simulink model "RPPPWM"  (R2014a)
settings: Solver=ode113  StartTime=0.0  StopTime=8  RelTol=1e-3
undefined symbols (not defined in the file): J, p, Rr, Rs, wb, Xlr, Xls, Xmstar
libraries: powerlib x16, simulink_extras x9, powerlib_extras x1
settings Model: Creator=afroz khan  LastModifiedBy=Divya M

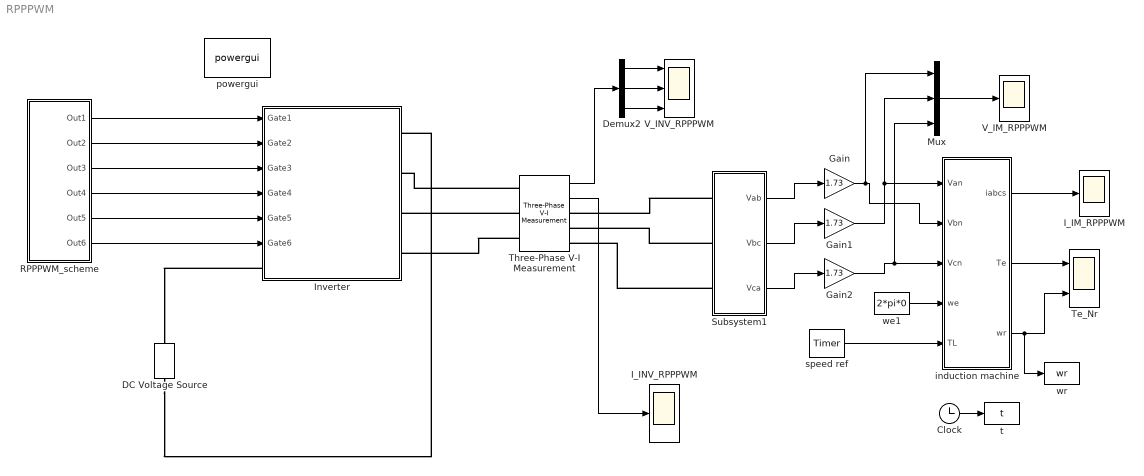
== system RPPPWM ==
  Clock : Clock
  DC Voltage Source : powerlib/Electrical Sources/DC Voltage Source  Amplitude=400  Measurements=None
  Demux2 : Demux  Outputs=3
  Gain : Gain  Gain=1.73
  Gain1 : Gain  Gain=1.73
  Gain2 : Gain  Gain=1.73
  I_IM_RPPPWM : Scope
      settings: YMin=-80  YMax=70  SaveName=I_IM_RPPPWM  MaxDataPoints=50000
  I_INV_RPPPWM : Scope
      settings: YMin=-75  YMax=75  SaveName=I_INV_RPPPWM  MaxDataPoints=50000
  Inverter : Subsystem
  Mux : Mux  Inputs=3
  RPPPWM_scheme : Subsystem
  Subsystem1 : Subsystem
  Te_Nr : Scope  NumInputPorts=2
      settings: TimeRange=1.5  YMin=-35~265  YMax=75~315  SaveName=ScopeData2
  Three-Phase V-I Measurement : powerlib/Measurements/Three-Phase V-I Measurement  VoltageMeasurement=phase-to-phase  SetLabelV=off  LabelV=Vabc  Vpu=off  VpuLL=off  CurrentMeasurement=yes  SetLabelI=off  LabelI=Iabc  Ipu=off  Pbase=100e6  Vbase=500e3  OutputType=Complex  PhasorSimulation=off  PSBequivalent=0
  V_IM_RPPPWM : Scope
      settings: YMin=-700  YMax=700  SaveName=V_IM_RPPPWM  MaxDataPoints=50000
  V_INV_RPPPWM : Scope  NumInputPorts=3
      settings: YMin=-225~-5~-5  YMax=225~5~5  SaveName=V_INV_RPPPWM  MaxDataPoints=50000
  "induction machine " : Subsystem
  powergui : powerlib/powergui  Priority=1  SimulationMode=Discrete  SolverType=Tustin  SampleTime=50e-6  frequency=60  SPID=off  DisableSnubberDevices=off  DisableRonSwitches=off  DisableVfSwitches=off  SwTol=0  Interpol=off  DisplayEquations=off  Ts=0  methode=off  frequencyindice=0  Pbase=100e6  ErrMax=1e-4  Iterations=50  UnitsV=kV  UnitsW=MW  FunctionMessages=off  echomessages=off  HookPort=off  EnableUseOfTLC=off  x0status=blocks  RestoreLinks=warning  ResistiveCurrentMeasurement=off  Frange=[0:2:500]  Ylog=off  Xlog=on  ShowGrid=off  save=off  variable=ZData  structure=V_IM_RPPPWM  ZoomFFT=off  StartTime=7.5  cycles=10  DisplayStyle=1  fundamental=50  FreqAxis=off  MaxFrequency=5000  frequencyindicesteady=1  RmsSteady=1  display=off
  speed ref : powerlib_extras/Control  Blocks/Timer  t=[ 0 1]  e=[10 10]
  t : ToWorkspace  VariableName=t  SampleTime=-1
  we1 : Constant  Value=2*pi*0
  wr : ToWorkspace  VariableName=wr  SampleTime=-1
  wires:
  RPPPWM_scheme/1(Out1) -> Inverter/1(Gate1)
  RPPPWM_scheme/2(Out2) -> Inverter/2(Gate2)
  RPPPWM_scheme/3(Out3) -> Inverter/3(Gate3)
  RPPPWM_scheme/4(Out4) -> Inverter/4(Gate4)
  RPPPWM_scheme/5(Out5) -> Inverter/5(Gate5)
  RPPPWM_scheme/6(Out6) -> Inverter/6(Gate6)
  Demux2/1 -> V_INV_RPPPWM/1
  Demux2/2 -> V_INV_RPPPWM/2
  Demux2/3 -> V_INV_RPPPWM/3
  Three-Phase V-I Measurement/1 -> Demux2/1
  Gain2/1 -> "induction machine "/3(Vcn), Mux/3
  Subsystem1/3(Vca) -> Gain2/1
  Gain1/1 -> "induction machine "/1(Van), Mux/2
  Gain/1 -> "induction machine "/2(Vbn), Mux/1
  Subsystem1/2(Vbc) -> Gain1/1
  Subsystem1/1(Vab) -> Gain/1
  Mux/1 -> V_IM_RPPPWM/1
  speed ref/1 -> "induction machine "/5(TL)
  we1/1 -> "induction machine "/4(we)
  "induction machine "/2(Te) -> Te_Nr/1
  "induction machine "/3(wr) -> wr/1, Te_Nr/2
  "induction machine "/1(iabcs) -> I_IM_RPPPWM/1
  Clock/1 -> t/1
  Three-Phase V-I Measurement/2 -> I_INV_RPPPWM/1
  connections:
  Inverter/LConn1 -- DC Voltage Source/RConn1
  DC Voltage Source/LConn1 -- Inverter/RConn1
  Three-Phase V-I Measurement/LConn1 -- Inverter/RConn2
  Three-Phase V-I Measurement/LConn2 -- Inverter/RConn3
  Three-Phase V-I Measurement/LConn3 -- Inverter/RConn4
  Subsystem1/LConn1 -- Three-Phase V-I Measurement/RConn1
  Subsystem1/LConn2 -- Three-Phase V-I Measurement/RConn2
  Subsystem1/LConn3 -- Three-Phase V-I Measurement/RConn3

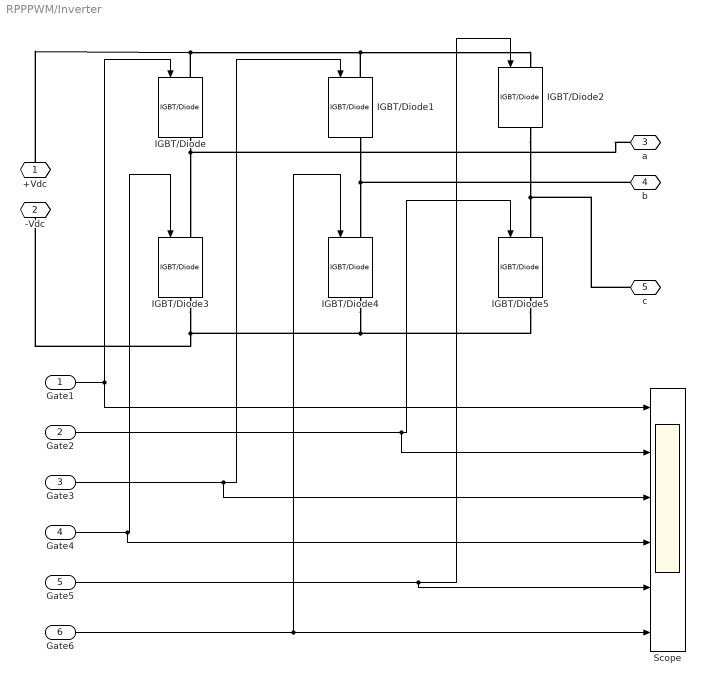
== system RPPPWM/Inverter ==
  Gate1 : Inport
  Gate2 : Inport  Port=2
  Gate3 : Inport  Port=3
  Gate4 : Inport  Port=4
  Gate5 : Inport  Port=5
  Gate6 : Inport  Port=6
  IGBT/Diode{,1..5} (6 alike) : powerlib/Power Electronics/IGBT//Diode  Ron=1e-3  Rs=1e5  Cs=inf  Measurements=on
  Scope : Scope  NumInputPorts=6
      settings: YMin=-5~-5~-5~-5~-5~-5  YMax=5~5~5~5~5~5
  +Vdc : PMIOPort  Port=1  Side=Left
  -Vdc : PMIOPort  Port=2  Side=Right
  a : PMIOPort  Port=3  Side=Right
  b : PMIOPort  Port=4  Side=Right
  c : PMIOPort  Port=5  Side=Right
  wires:
  Gate2/1 -> Scope/2, IGBT/Diode5/1
  Gate3/1 -> Scope/3, IGBT/Diode1/1
  Gate4/1 -> Scope/4, IGBT/Diode3/1
  Gate6/1 -> IGBT/Diode4/1, Scope/6
  Gate1/1 -> IGBT/Diode/1, Scope/1
  Gate5/1 -> Scope/5, IGBT/Diode2/1
  connections:
  IGBT/Diode5/RConn1 -- IGBT/Diode4/RConn1 -- -Vdc/RConn1 -- IGBT/Diode3/RConn1
  IGBT/Diode2/RConn1 -- c/RConn1 -- IGBT/Diode5/LConn1
  IGBT/Diode1/RConn1 -- b/RConn1 -- IGBT/Diode4/LConn1
  IGBT/Diode/LConn1 -- +Vdc/RConn1 -- IGBT/Diode1/LConn1 -- IGBT/Diode2/LConn1
  IGBT/Diode/RConn1 -- a/RConn1 -- IGBT/Diode3/LConn1

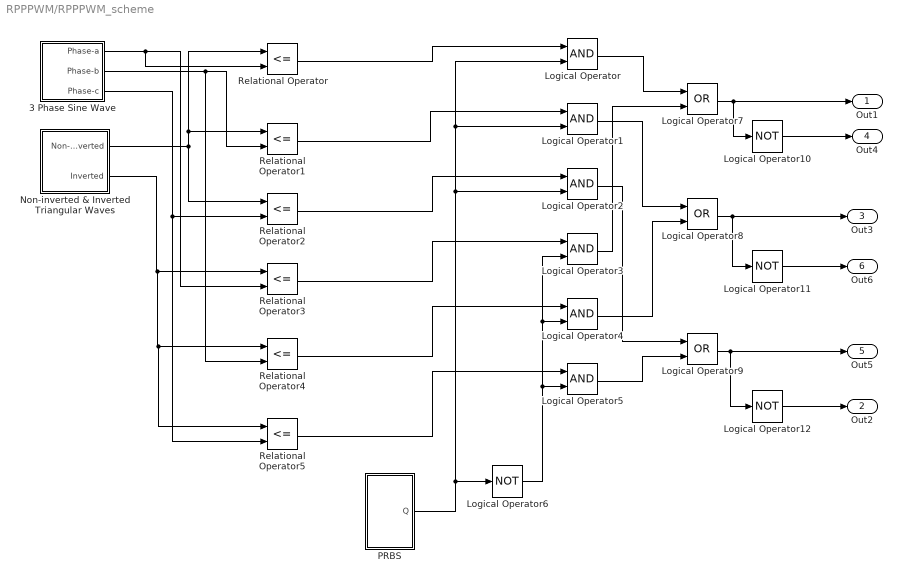
== system RPPPWM/RPPPWM_scheme ==
  3 Phase Sine Wave : Subsystem
  Logical Operator{,1..5} (6 alike) : Logic  AllPortsSameDT=off  OutDataTypeStr=boolean
  Logical Operator{6,10..12} (4 alike) : Logic  Operator=NOT  AllPortsSameDT=off  OutDataTypeStr=boolean
  Logical Operator7 : Logic  Operator=OR  AllPortsSameDT=off  OutDataTypeStr=boolean
  Logical Operator8 : Logic  Operator=OR  AllPortsSameDT=off  OutDataTypeStr=boolean
  Logical Operator9 : Logic  Operator=OR  AllPortsSameDT=off  OutDataTypeStr=boolean
  Non-inverted & Inverted Triangular Waves : Subsystem
  PRBS : Subsystem
  Relational Operator{,1..5} (6 alike) : RelationalOperator  Operator=<=  OutDataTypeStr=boolean
  Out1 : Outport
  Out2 : Outport  Port=2
  Out3 : Outport  Port=3
  Out4 : Outport  Port=4
  Out5 : Outport  Port=5
  Out6 : Outport  Port=6
  wires:
  Non-inverted & Inverted Triangular Waves/1(Non-inverted) -> Relational Operator2/1, Relational Operator1/1, Relational Operator/1
  Non-inverted & Inverted Triangular Waves/2(Inverted) -> Relational Operator5/1, Relational Operator4/1, Relational Operator3/1
  3 Phase Sine Wave/1("\tPhase-a") -> Relational Operator3/2, Relational Operator/2
  3 Phase Sine Wave/2(Phase-b) -> Relational Operator4/2, Relational Operator1/2
  3 Phase Sine Wave/3(Phase-c) -> Relational Operator5/2, Relational Operator2/2
  Relational Operator/1 -> Logical Operator/1
  Relational Operator1/1 -> Logical Operator1/1
  Relational Operator2/1 -> Logical Operator2/1
  Relational Operator3/1 -> Logical Operator3/1
  Relational Operator4/1 -> Logical Operator4/1
  Relational Operator5/1 -> Logical Operator5/1
  PRBS/1(Q) -> Logical Operator6/1, Logical Operator2/2, Logical Operator1/2, Logical Operator/2
  Logical Operator6/1 -> Logical Operator5/2, Logical Operator4/2, Logical Operator3/2
  Logical Operator/1 -> Logical Operator7/1
  Logical Operator1/1 -> Logical Operator8/1
  Logical Operator2/1 -> Logical Operator9/1
  Logical Operator3/1 -> Logical Operator7/2
  Logical Operator4/1 -> Logical Operator8/2
  Logical Operator5/1 -> Logical Operator9/2
  Logical Operator7/1 -> Logical Operator10/1, Out1/1
  Logical Operator8/1 -> Logical Operator11/1, Out3/1
  Logical Operator9/1 -> Logical Operator12/1, Out5/1
  Logical Operator10/1 -> Out4/1
  Logical Operator11/1 -> Out6/1
  Logical Operator12/1 -> Out2/1

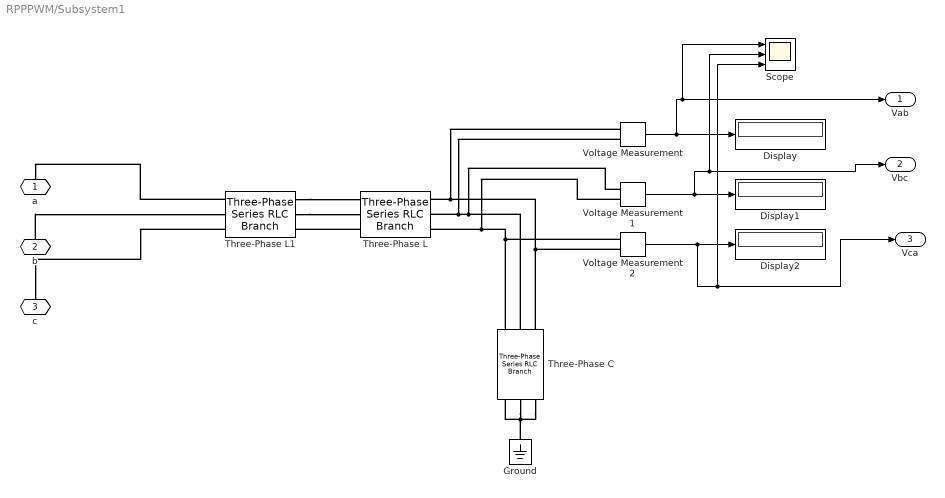
== system RPPPWM/Subsystem1 ==
  Display : Display
  Display1 : Display
  Display2 : Display
  Ground : powerlib/Elements/Ground  LConnTagsString=a
  Scope : Scope  NumInputPorts=3
      settings: YMin=-200~-200~-200  YMax=200~200~200  SaveName=ScopeData3
  "Three-Phase C " : powerlib/Elements/Three-Phase Series RLC Branch  LConnTagsString=A|B|C  RConnTagsString=A|B|C  BranchType=C  Resistance=1  Inductance=10  Capacitance=0.2420e-3  Measurements=None
  Three-Phase L : powerlib/Elements/Three-Phase Series RLC Branch  LConnTagsString=A|B|C  RConnTagsString=A|B|C  BranchType=L  Resistance=1  Inductance=0.0150e-2  Capacitance=1e-6  Measurements=None
  Three-Phase L1 : powerlib/Elements/Three-Phase Series RLC Branch  LConnTagsString=A|B|C  RConnTagsString=A|B|C  BranchType=R  Resistance=15  Inductance=1e-1  Capacitance=1e-6  Measurements=None
  Voltage Measurement : powerlib/Measurements/Voltage Measurement  PhasorSimulation=off  OutputType=Complex  PSBequivalent=0
  Voltage Measurement1 : powerlib/Measurements/Voltage Measurement  PhasorSimulation=off  OutputType=Complex  PSBequivalent=0
  Voltage Measurement2 : powerlib/Measurements/Voltage Measurement  PhasorSimulation=off  OutputType=Complex  PSBequivalent=0
  a : PMIOPort  Port=1  Side=Left
  b : PMIOPort  Port=2  Side=Left
  c : PMIOPort  Port=3  Side=Left
  Vab : Outport
  Vbc : Outport  Port=2
  Vca : Outport  Port=3
  wires:
  Voltage Measurement/1 -> Scope/1, Vab/1, Display/1
  Voltage Measurement1/1 -> Scope/2, Vbc/1, Display1/1
  Voltage Measurement2/1 -> Scope/3, Vca/1, Display2/1
  connections:
  "Three-Phase C "/LConn1 -- Voltage Measurement2/LConn1 -- Voltage Measurement1/LConn2 -- Three-Phase L/RConn3
  "Three-Phase C "/LConn2 -- Voltage Measurement1/LConn1 -- Voltage Measurement/LConn2 -- Three-Phase L/RConn2
  "Three-Phase C "/LConn3 -- Voltage Measurement2/LConn2 -- Voltage Measurement/LConn1 -- Three-Phase L/RConn1
  Ground/LConn1 -- "Three-Phase C "/RConn2 -- "Three-Phase C "/RConn1 -- "Three-Phase C "/RConn3
  Three-Phase L1/RConn1 -- Three-Phase L/LConn1
  Three-Phase L1/RConn2 -- Three-Phase L/LConn2
  Three-Phase L/LConn3 -- Three-Phase L1/RConn3
  Three-Phase L1/LConn1 -- a/RConn1
  b/RConn1 -- Three-Phase L1/LConn2
  Three-Phase L1/LConn3 -- c/RConn1

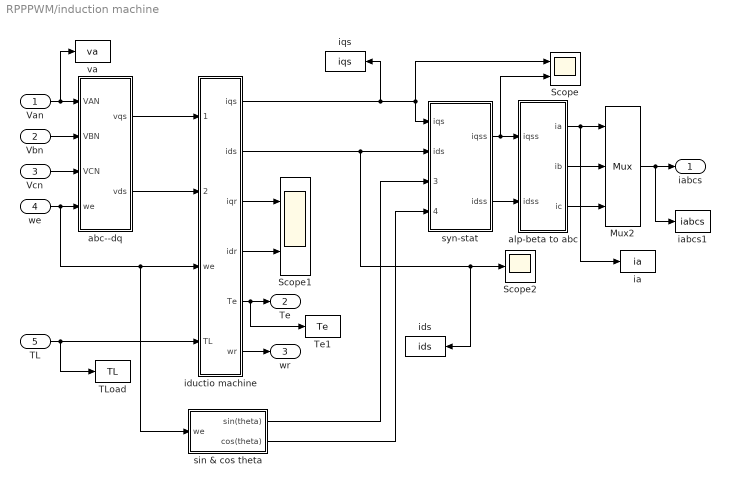
== system RPPPWM/induction machine  ==
  Van : Inport
  Vbn : Inport  Port=2
  Vcn : Inport  Port=3
  we : Inport  Port=4
  TL : Inport  Port=5
  " alp-beta to abc" : Subsystem
  Mux2 : Mux  Inputs=3
  Scope : Scope  NumInputPorts=2
      settings: YMin=-60~-5  YMax=50~5  SaveName=ScopeData11
  Scope1 : Scope  NumInputPorts=2
      settings: TimeRange=0.25  YMin=-350~-5  YMax=350~5  SampleInput=on
  Scope2 : Scope
      settings: YMin=-60  YMax=50  SaveName=ScopeData12
  TLoad : ToWorkspace  VariableName=TL  SampleTime=-1
  Te1 : ToWorkspace  VariableName=Te  SampleTime=-1
  "abc--dq " : Subsystem
  ia : ToWorkspace  VariableName=ia  SampleTime=-1
  iabcs1 : ToWorkspace  VariableName=iabcs  SampleTime=-1
  ids : ToWorkspace  VariableName=ids  SampleTime=-1
  iductio machine : Subsystem
  iqs : ToWorkspace  VariableName=iqs  SampleTime=-1
  sin & cos theta : Subsystem
  syn-stat : Subsystem
  va : ToWorkspace  VariableName=va  SampleTime=-1
  iabcs : Outport
  Te : Outport  Port=2
  wr : Outport  Port=3
  wires:
  Van/1 -> "abc--dq "/1(VAN), va/1
  Vbn/1 -> "abc--dq "/2(VBN)
  Vcn/1 -> "abc--dq "/3(VCN)
  we/1 -> sin & cos theta/1(we), iductio machine/3(we), "abc--dq "/4(we)
  TL/1 -> iductio machine/4(TL), TLoad/1
  iductio machine/4(idr) -> Scope1/2
  iductio machine/3(iqr) -> Scope1/1
  sin & cos theta/2(cos(theta)) -> syn-stat/4(cos(theta))
  sin & cos theta/1(sin(theta)) -> syn-stat/3(sin(theta))
  " alp-beta to abc"/3(ic) -> Mux2/3
  " alp-beta to abc"/2(ib) -> Mux2/2
  syn-stat/2(idss) -> " alp-beta to abc"/2(idss)
  syn-stat/1(iqss) -> " alp-beta to abc"/1(iqss), Scope/2
  iductio machine/1(iqs) -> syn-stat/1(iqs), Scope/1, iqs/1
  "abc--dq "/2(vds) -> iductio machine/2(vds)
  "abc--dq "/1(vqs) -> iductio machine/1(vqs)
  iductio machine/5(Te) -> Te/1, Te1/1
  iductio machine/2(ids) -> syn-stat/2(ids), Scope2/1, ids/1
  " alp-beta to abc"/1(ia) -> Mux2/1, ia/1
  Mux2/1 -> iabcs/1, iabcs1/1
  iductio machine/6(wr) -> wr/1

== system RPPPWM/RPPPWM_scheme/3 Phase Sine Wave ==
  Scope : Scope  NumInputPorts=3
      settings: YMin=-5~-5~-5  YMax=5~5~5  SaveName=ScopeData9
  Sine Wave : Sin  Amplitude=0.8  Frequency=314  SampleTime=0
  Sine Wave1 : Sin  Amplitude=0.8  Frequency=314  Phase=(2*pi)/3  SampleTime=0
  Sine Wave2 : Sin  Amplitude=0.8  Frequency=314  Phase=(4*pi)/3  SampleTime=0
  "\tPhase-a" : Outport
  Phase-b : Outport  Port=2
  Phase-c : Outport  Port=3
  wires:
  Sine Wave1/1 -> Scope/2, Phase-b/1
  Sine Wave/1 -> Scope/1, "\tPhase-a"/1
  Sine Wave2/1 -> Scope/3, Phase-c/1

== system RPPPWM/RPPPWM_scheme/Non-inverted & Inverted Triangular Waves ==
  note: Triangular Wave
  Constant : Constant  Value=-1
  Dot Product : DotProduct  InputSameDT=on  OutDataTypeStr=Inherit: Inherit via internal rule
  Integrator : Integrator
  Pulse Generator : DiscretePulseGenerator  PulseType=Time based  Amplitude=12000  Period=1e-3/3  PulseWidth=50
  Pulse Generator1 : DiscretePulseGenerator  PulseType=Time based  Amplitude=-12000  Period=1/3e3  PulseWidth=50  PhaseDelay=1/6e3
  Scope : Scope  NumInputPorts=2
      settings: YMin=-2.5~-37.5  YMax=37.5~2.5  SaveName=ScopeData6
  Sum : Sum  Inputs=|++
  Sum1 : Sum  Inputs=|++
  Non-inverted : Outport
  Inverted : Outport  Port=2
  wires:
  Dot Product/1 -> Scope/2, Inverted/1  "Inverted Triangular Wave"
  Pulse Generator/1 -> Sum/1
  Pulse Generator1/1 -> Sum/2
  Sum/1 -> Integrator/1
  Sum1/1 -> Scope/1, Non-inverted/1, Dot Product/1
  Constant/1 -> Dot Product/2, Sum1/2
  Integrator/1 -> Sum1/1

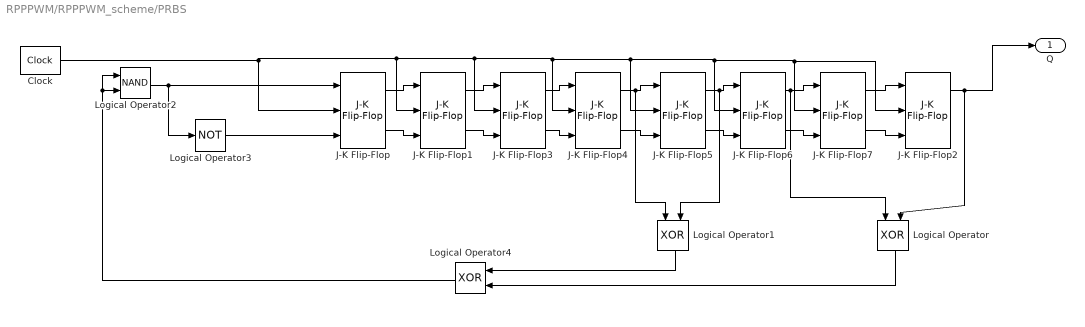
== system RPPPWM/RPPPWM_scheme/PRBS ==
  Clock : simulink_extras/Flip Flops/Clock  period=1/3e3
  J-K Flip-Flop{,1..7} (8 alike) : simulink_extras/Flip Flops/J-K Flip-Flop  initial_condition=0
  Logical Operator : Logic  Operator=XOR  AllPortsSameDT=off  OutDataTypeStr=boolean
  Logical Operator1 : Logic  Operator=XOR  AllPortsSameDT=off  OutDataTypeStr=boolean
  Logical Operator2 : Logic  Operator=NAND  AllPortsSameDT=off  OutDataTypeStr=boolean
  Logical Operator3 : Logic  Operator=NOT  AllPortsSameDT=off  OutDataTypeStr=boolean
  Logical Operator4 : Logic  Operator=XOR  AllPortsSameDT=off  OutDataTypeStr=boolean
  Q : Outport
  wires:
  J-K Flip-Flop6/1 -> Logical Operator/1, J-K Flip-Flop7/1
  Logical Operator2/1 -> Logical Operator3/1, J-K Flip-Flop/1
  J-K Flip-Flop5/2 -> J-K Flip-Flop6/3
  J-K Flip-Flop3/2 -> J-K Flip-Flop4/3
  Logical Operator/1 -> Logical Operator4/2
  J-K Flip-Flop7/1 -> J-K Flip-Flop2/1
  J-K Flip-Flop5/1 -> J-K Flip-Flop6/1, Logical Operator1/2
  Logical Operator1/1 -> Logical Operator4/1
  J-K Flip-Flop1/2 -> J-K Flip-Flop3/3
  J-K Flip-Flop/2 -> J-K Flip-Flop1/3
  Logical Operator4/1 -> Logical Operator2/2, Logical Operator2/1
  J-K Flip-Flop3/1 -> J-K Flip-Flop4/1
  J-K Flip-Flop4/1 -> J-K Flip-Flop5/1, Logical Operator1/1
  J-K Flip-Flop7/2 -> J-K Flip-Flop2/3
  J-K Flip-Flop6/2 -> J-K Flip-Flop7/3
  J-K Flip-Flop2/1 -> Q/1, Logical Operator/2
  Logical Operator3/1 -> J-K Flip-Flop/3
  Clock/1 -> J-K Flip-Flop3/2, J-K Flip-Flop2/2, J-K Flip-Flop7/2, J-K Flip-Flop6/2, J-K Flip-Flop5/2, J-K Flip-Flop4/2, J-K Flip-Flop1/2, J-K Flip-Flop/2
  J-K Flip-Flop4/2 -> J-K Flip-Flop5/3
  J-K Flip-Flop/1 -> J-K Flip-Flop1/1
  J-K Flip-Flop1/1 -> J-K Flip-Flop3/1

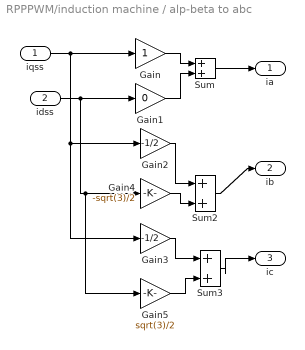
== system RPPPWM/induction machine / alp-beta to abc ==
  iqss : Inport
  idss : Inport  Port=2
  Gain : Gain  SaturateOnIntegerOverflow=on  OutDataTypeStr=Inherit: Same as input  ParamDataTypeStr=Inherit: Same as input
  Gain1 : Gain  Gain=0  SaturateOnIntegerOverflow=on  OutDataTypeStr=Inherit: Same as input  ParamDataTypeStr=Inherit: Same as input
  Gain2 : Gain  Gain=-1/2  SaturateOnIntegerOverflow=on  OutDataTypeStr=Inherit: Same as input  ParamDataTypeStr=Inherit: Same as input
  Gain3 : Gain  Gain=-1/2  SaturateOnIntegerOverflow=on  OutDataTypeStr=Inherit: Same as input  ParamDataTypeStr=Inherit: Same as input
  Gain4 : Gain  Gain=-sqrt(3)/2  SaturateOnIntegerOverflow=on  OutDataTypeStr=Inherit: Same as input  ParamDataTypeStr=Inherit: Same as input
  Gain5 : Gain  Gain=sqrt(3)/2  SaturateOnIntegerOverflow=on  OutDataTypeStr=Inherit: Same as input  ParamDataTypeStr=Inherit: Same as input
  Sum : Sum  Inputs=|++  SaturateOnIntegerOverflow=on
  Sum2 : Sum  Inputs=|++  SaturateOnIntegerOverflow=on
  Sum3 : Sum  Inputs=|++  SaturateOnIntegerOverflow=on
  ia : Outport
  ib : Outport  Port=2
  ic : Outport  Port=3
  wires:
  Gain/1 -> Sum/1
  Gain1/1 -> Sum/2
  Gain2/1 -> Sum2/1
  Gain4/1 -> Sum2/2
  Gain3/1 -> Sum3/1
  Gain5/1 -> Sum3/2
  iqss/1 -> Gain3/1, Gain2/1, Gain/1
  idss/1 -> Gain5/1, Gain4/1, Gain1/1
  Sum3/1 -> ic/1
  Sum2/1 -> ib/1
  Sum/1 -> ia/1

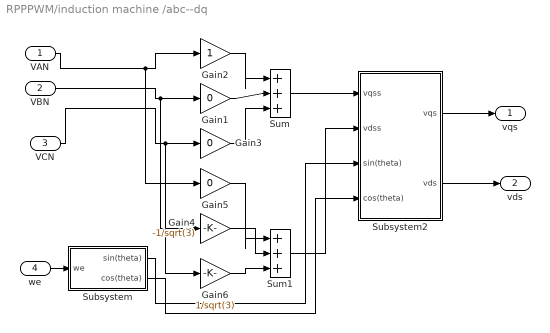
== system RPPPWM/induction machine /abc--dq  ==
  VAN : Inport
  VBN : Inport  Port=2
  VCN : Inport  Port=3
  we : Inport  Port=4
  Gain1 : Gain  Gain=0  SaturateOnIntegerOverflow=on  OutDataTypeStr=Inherit: Same as input  ParamDataTypeStr=Inherit: Same as input
  Gain2 : Gain  SaturateOnIntegerOverflow=on  OutDataTypeStr=Inherit: Same as input  ParamDataTypeStr=Inherit: Same as input
  Gain3 : Gain  Gain=0  SaturateOnIntegerOverflow=on  OutDataTypeStr=Inherit: Same as input  ParamDataTypeStr=Inherit: Same as input
  Gain4 : Gain  Gain=-1/sqrt(3)  SaturateOnIntegerOverflow=on  OutDataTypeStr=Inherit: Same as input  ParamDataTypeStr=Inherit: Same as input
  Gain5 : Gain  Gain=0  SaturateOnIntegerOverflow=on  OutDataTypeStr=Inherit: Same as input  ParamDataTypeStr=Inherit: Same as input
  Gain6 : Gain  Gain=1/sqrt(3)  SaturateOnIntegerOverflow=on  OutDataTypeStr=Inherit: Same as input  ParamDataTypeStr=Inherit: Same as input
  Subsystem : Subsystem
  Subsystem2 : Subsystem
  Sum : Sum  Inputs=|+++  SaturateOnIntegerOverflow=on
  Sum1 : Sum  Inputs=|+++  SaturateOnIntegerOverflow=on
  vqs : Outport
  vds : Outport  Port=2
  wires:
  Gain2/1 -> Sum/1
  Gain1/1 -> Sum/2
  Gain3/1 -> Sum/3
  Gain5/1 -> Sum1/1
  Gain4/1 -> Sum1/2
  Gain6/1 -> Sum1/3
  Sum/1 -> Subsystem2/1(vqss)
  Sum1/1 -> Subsystem2/2(vdss)
  VAN/1 -> Gain2/1, Gain5/1
  VBN/1 -> Gain1/1, Gain4/1
  VCN/1 -> Gain3/1, Gain6/1
  Subsystem2/1(vqs) -> vqs/1
  Subsystem2/2(vds) -> vds/1
  we/1 -> Subsystem/1(we)
  Subsystem/1(sin(theta)) -> Subsystem2/3(sin(theta))
  Subsystem/2(cos(theta)) -> Subsystem2/4(cos(theta))

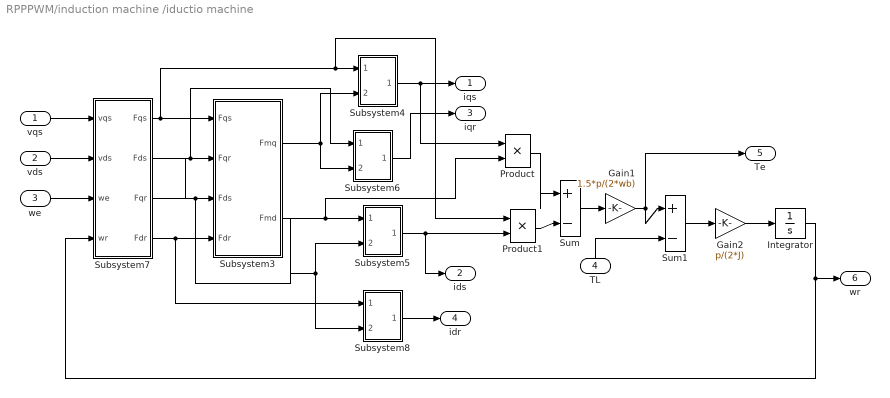
== system RPPPWM/induction machine /iductio machine ==
  vqs : Inport
  vds : Inport  Port=2
  we : Inport  Port=3
  TL : Inport  Port=4
  Gain1 : Gain  Gain=1.5*p/(2*wb)  SaturateOnIntegerOverflow=on  OutDataTypeStr=Inherit: Same as input  ParamDataTypeStr=Inherit: Same as input
  Gain2 : Gain  Gain=p/(2*J)  SaturateOnIntegerOverflow=on  OutDataTypeStr=Inherit: Same as input  ParamDataTypeStr=Inherit: Same as input
  Integrator : Integrator
  Product : Product  SaturateOnIntegerOverflow=on  OutDataTypeStr=Inherit: Same as first input
  Product1 : Product  SaturateOnIntegerOverflow=on  OutDataTypeStr=Inherit: Same as first input
  Subsystem3 : Subsystem
  Subsystem4 : Subsystem
  Subsystem5 : Subsystem
  Subsystem6 : Subsystem
  Subsystem7 : Subsystem
  Subsystem8 : Subsystem
  Sum : Sum  Inputs=|+-  SaturateOnIntegerOverflow=on
  Sum1 : Sum  Inputs=|+-  SaturateOnIntegerOverflow=on
  iqs : Outport
  ids : Outport  Port=2
  iqr : Outport  Port=3
  idr : Outport  Port=4
  Te : Outport  Port=5
  wr : Outport  Port=6
  wires:
  Subsystem7/1(Fqs) -> Subsystem3/1(Fqs), Subsystem4/1(Fqs), Product1/1
  Subsystem3/1(Fmq) -> Subsystem4/2(Fmq), Subsystem6/2(Fmq)
  Subsystem3/2(Fmd) -> Subsystem5/2(Fmd), Subsystem8/2(Fmd)
  Subsystem4/1(iqs) -> Product/1, iqs/1
  Subsystem5/1(ids) -> Product1/2, ids/1
  Sum/1 -> Gain1/1
  Gain1/1 -> Te/1, Sum1/1
  Gain2/1 -> Integrator/1
  Integrator/1 -> wr/1, Subsystem7/4(wr)
  we/1 -> Subsystem7/3(we)
  vqs/1 -> Subsystem7/1(vqs)
  vds/1 -> Subsystem7/2(vds)
  Subsystem6/1(iqr) -> iqr/1
  Subsystem8/1(idr) -> idr/1
  Product1/1 -> Sum/2
  Product/1 -> Sum/1
  Sum1/1 -> Gain2/1
  TL/1 -> Sum1/2
  Subsystem7/3(Fqr) -> Subsystem3/2(Fqr), Subsystem6/1(Fqr)
  Subsystem7/4(Fdr) -> Subsystem3/4(Fdr), Subsystem8/1(Fdr)
  Subsystem7/2(Fds) -> Subsystem3/3(Fds), Subsystem5/1(Fds), Product/2

== system RPPPWM/induction machine /sin & cos theta ==
  we : Inport
  Integrator : Integrator
  Trigonometric Function : Trigonometry
  Trigonometric Function1 : Trigonometry  Operator=cos
  sin(theta) : Outport
  cos(theta) : Outport  Port=2
  wires:
  Integrator/1 -> Trigonometric Function/1, Trigonometric Function1/1
  Trigonometric Function/1 -> sin(theta)/1
  we/1 -> Integrator/1
  Trigonometric Function1/1 -> cos(theta)/1

== system RPPPWM/induction machine /syn-stat ==
  iqs : Inport
  ids : Inport  Port=2
  sin(theta) : Inport  Port=3
  cos(theta) : Inport  Port=4
  Product{,1..3} (4 alike) : Product  SaturateOnIntegerOverflow=on  OutDataTypeStr=Inherit: Same as first input
  Sum1 : Sum  SaturateOnIntegerOverflow=on
  Sum4 : Sum  Inputs=-+  SaturateOnIntegerOverflow=on
  iqss : Outport
  idss : Outport  Port=2
  wires:
  ids/1 -> Product3/1, Product/1
  iqs/1 -> Product2/1, Product1/1
  Product1/1 -> Sum1/1
  Product/1 -> Sum1/2
  Product2/1 -> Sum4/1
  Product3/1 -> Sum4/2
  sin(theta)/1 -> Product/2, Product2/2
  cos(theta)/1 -> Product1/2, Product3/2
  Sum1/1 -> iqss/1
  Sum4/1 -> idss/1

== system RPPPWM/induction machine /abc--dq /Subsystem ==
  we : Inport
  Integrator : Integrator
  Trigonometric Function : Trigonometry
  Trigonometric Function1 : Trigonometry  Operator=cos
  sin(theta) : Outport
  cos(theta) : Outport  Port=2
  wires:
  Integrator/1 -> Trigonometric Function/1, Trigonometric Function1/1
  Trigonometric Function/1 -> sin(theta)/1
  we/1 -> Integrator/1
  Trigonometric Function1/1 -> cos(theta)/1

== system RPPPWM/induction machine /abc--dq /Subsystem2 ==
  vqss : Inport
  vdss : Inport  Port=2
  sin(theta) : Inport  Port=3
  cos(theta) : Inport  Port=4
  Product{,1..3} (4 alike) : Product  SaturateOnIntegerOverflow=on  OutDataTypeStr=Inherit: Same as first input
  Sum : Sum  Inputs=+-  SaturateOnIntegerOverflow=on
  Sum1 : Sum  SaturateOnIntegerOverflow=on
  vqs : Outport
  vds : Outport  Port=2
  wires:
  vqss/1 -> Product2/1, Product/1
  vdss/1 -> Product1/1, Product3/1
  sin(theta)/1 -> Product2/2, Product1/2
  Product/1 -> Sum/1
  Product1/1 -> Sum/2
  Product2/1 -> Sum1/1
  Product3/1 -> Sum1/2
  Sum/1 -> vqs/1
  Sum1/1 -> vds/1
  cos(theta)/1 -> Product3/2, Product/2

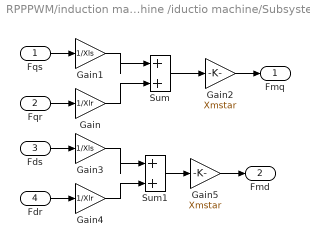
== system RPPPWM/induction machine /iductio machine/Subsystem3 ==
  Fqs : Inport
  Fqr : Inport  Port=2
  Fds : Inport  Port=3
  Fdr : Inport  Port=4
  Gain : Gain  Gain=1/Xlr  SaturateOnIntegerOverflow=on  OutDataTypeStr=Inherit: Same as input  ParamDataTypeStr=Inherit: Same as input
  Gain1 : Gain  Gain=1/Xls  SaturateOnIntegerOverflow=on  OutDataTypeStr=Inherit: Same as input  ParamDataTypeStr=Inherit: Same as input
  Gain2 : Gain  Gain=Xmstar  SaturateOnIntegerOverflow=on  OutDataTypeStr=Inherit: Same as input  ParamDataTypeStr=Inherit: Same as input
  Gain3 : Gain  Gain=1/Xls  SaturateOnIntegerOverflow=on  OutDataTypeStr=Inherit: Same as input  ParamDataTypeStr=Inherit: Same as input
  Gain4 : Gain  Gain=1/Xlr  SaturateOnIntegerOverflow=on  OutDataTypeStr=Inherit: Same as input  ParamDataTypeStr=Inherit: Same as input
  Gain5 : Gain  Gain=Xmstar  SaturateOnIntegerOverflow=on  OutDataTypeStr=Inherit: Same as input  ParamDataTypeStr=Inherit: Same as input
  Sum : Sum  Inputs=|++  SaturateOnIntegerOverflow=on
  Sum1 : Sum  Inputs=|++  SaturateOnIntegerOverflow=on
  Fmq : Outport
  Fmd : Outport  Port=2
  wires:
  Gain1/1 -> Sum/1
  Gain/1 -> Sum/2
  Sum/1 -> Gain2/1
  Gain3/1 -> Sum1/1
  Gain4/1 -> Sum1/2
  Sum1/1 -> Gain5/1
  Fqs/1 -> Gain1/1
  Gain2/1 -> Fmq/1
  Fqr/1 -> Gain/1
  Fds/1 -> Gain3/1
  Gain5/1 -> Fmd/1
  Fdr/1 -> Gain4/1

== system RPPPWM/induction machine /iductio machine/Subsystem4 ==
  Fqs : Inport
  Fmq : Inport  Port=2
  Gain2 : Gain  Gain=1/Xls  SaturateOnIntegerOverflow=on  OutDataTypeStr=Inherit: Same as input  ParamDataTypeStr=Inherit: Same as input
  Sum : Sum  Inputs=|+-  SaturateOnIntegerOverflow=on
  iqs : Outport
  wires:
  Sum/1 -> Gain2/1
  Fqs/1 -> Sum/1
  Gain2/1 -> iqs/1
  Fmq/1 -> Sum/2

== system RPPPWM/induction machine /iductio machine/Subsystem5 ==
  Fds : Inport
  Fmd : Inport  Port=2
  Gain2 : Gain  Gain=1/Xls  SaturateOnIntegerOverflow=on  OutDataTypeStr=Inherit: Same as input  ParamDataTypeStr=Inherit: Same as input
  Sum : Sum  Inputs=|+-  SaturateOnIntegerOverflow=on
  ids : Outport
  wires:
  Fmd/1 -> Sum/2
  Gain2/1 -> ids/1
  Fds/1 -> Sum/1
  Sum/1 -> Gain2/1

== system RPPPWM/induction machine /iductio machine/Subsystem6 ==
  Fqr : Inport
  Fmq : Inport  Port=2
  Gain2 : Gain  Gain=1/Xlr  SaturateOnIntegerOverflow=on  OutDataTypeStr=Inherit: Same as input  ParamDataTypeStr=Inherit: Same as input
  Sum : Sum  Inputs=|+-  SaturateOnIntegerOverflow=on
  iqr : Outport
  wires:
  Sum/1 -> Gain2/1
  Fqr/1 -> Sum/1
  Gain2/1 -> iqr/1
  Fmq/1 -> Sum/2

== system RPPPWM/induction machine /iductio machine/Subsystem7 ==
  vqs : Inport
  vds : Inport  Port=2
  we : Inport  Port=3
  wr : Inport  Port=4
  Subsystem3 : Subsystem
  Subsystem4 : Subsystem
  Subsystem5 : Subsystem
  Subsystem6 : Subsystem
  Fqs : Outport
  Fds : Outport  Port=2
  Fqr : Outport  Port=3
  Fdr : Outport  Port=4
  wires:
  vds/1 -> Subsystem4/1(vds)
  Subsystem3/1(Fqs) -> Fqs/1, Subsystem4/3(Fqs), Subsystem5/3(Fqs)
  Subsystem4/1(Fds) -> Subsystem3/3(Fds), Subsystem6/3(Fds), Fds/1
  Subsystem5/1(Fqr) -> Subsystem6/2(Fqr), Subsystem3/4(Fqr), Fqr/1
  Subsystem6/1(Fdr) -> Subsystem5/2(Fdr), Subsystem4/4(Fdr), Fdr/1
  wr/1 -> Subsystem5/4(wr), Subsystem6/4(wr)
  we/1 -> Subsystem3/2(we), Subsystem4/2(we), Subsystem5/1(we), Subsystem6/1(we)
  vqs/1 -> Subsystem3/1(vqs)

== system RPPPWM/induction machine /iductio machine/Subsystem8 ==
  Fdr : Inport
  Fmd : Inport  Port=2
  Gain2 : Gain  Gain=1/Xlr  SaturateOnIntegerOverflow=on  OutDataTypeStr=Inherit: Same as input  ParamDataTypeStr=Inherit: Same as input
  Sum : Sum  Inputs=|+-  SaturateOnIntegerOverflow=on
  idr : Outport
  wires:
  Fmd/1 -> Sum/2
  Gain2/1 -> idr/1
  Fdr/1 -> Sum/1
  Sum/1 -> Gain2/1

== system RPPPWM/induction machine /iductio machine/Subsystem7/Subsystem3 ==
  vqs : Inport
  we : Inport  Port=2
  Fds : Inport  Port=3
  Fqr : Inport  Port=4
  Integrator : Integrator  InitialCondition=0.00001
  Product : Product  SaturateOnIntegerOverflow=on  OutDataTypeStr=Inherit: Same as first input
  Sum : Sum  Inputs=+-+  SaturateOnIntegerOverflow=on
  Sum1 : Sum  SaturateOnIntegerOverflow=on
  wb : Gain  Gain=1/wb  SaturateOnIntegerOverflow=on  OutDataTypeStr=Inherit: Same as input  ParamDataTypeStr=Inherit: Same as input
  xmstar/xlr : Gain  Gain=Xmstar/Xlr  SaturateOnIntegerOverflow=on  OutDataTypeStr=Inherit: Same as input  ParamDataTypeStr=Inherit: Same as input
  xmstar/xlr1 : Gain  Gain=Rs/Xls  SaturateOnIntegerOverflow=on  OutDataTypeStr=Inherit: Same as input  ParamDataTypeStr=Inherit: Same as input
  xmstar/xlr2 : Gain  Gain=wb  SaturateOnIntegerOverflow=on  OutDataTypeStr=Inherit: Same as input  ParamDataTypeStr=Inherit: Same as input
  xmstar/xlr3 : Gain  Gain=(Xmstar/Xls)-1  SaturateOnIntegerOverflow=on  OutDataTypeStr=Inherit: Same as input  ParamDataTypeStr=Inherit: Same as input
  Fqs : Outport
  wires:
  wb/1 -> Product/1
  Product/1 -> Sum/2
  xmstar/xlr/1 -> Sum1/1
  Sum1/1 -> xmstar/xlr1/1
  Sum/1 -> xmstar/xlr2/1
  xmstar/xlr2/1 -> Integrator/1
  Integrator/1 -> xmstar/xlr3/1, Fqs/1
  xmstar/xlr3/1 -> Sum1/2
  we/1 -> wb/1
  vqs/1 -> Sum/1
  Fds/1 -> Product/2
  Fqr/1 -> xmstar/xlr/1
  xmstar/xlr1/1 -> Sum/3

== system RPPPWM/induction machine /iductio machine/Subsystem7/Subsystem4 ==
  vds : Inport
  we : Inport  Port=2
  Fqs : Inport  Port=3
  Fdr : Inport  Port=4
  Integrator : Integrator  InitialCondition=0.00001
  Product : Product  SaturateOnIntegerOverflow=on  OutDataTypeStr=Inherit: Same as first input
  Sum : Sum  Inputs=+++  SaturateOnIntegerOverflow=on
  Sum1 : Sum  SaturateOnIntegerOverflow=on
  wb : Gain  Gain=1/wb  SaturateOnIntegerOverflow=on  OutDataTypeStr=Inherit: Same as input  ParamDataTypeStr=Inherit: Same as input
  xmstar/xlr : Gain  Gain=Xmstar/Xlr  SaturateOnIntegerOverflow=on  OutDataTypeStr=Inherit: Same as input  ParamDataTypeStr=Inherit: Same as input
  xmstar/xlr1 : Gain  Gain=Rs/Xls  SaturateOnIntegerOverflow=on  OutDataTypeStr=Inherit: Same as input  ParamDataTypeStr=Inherit: Same as input
  xmstar/xlr2 : Gain  Gain=wb  SaturateOnIntegerOverflow=on  OutDataTypeStr=Inherit: Same as input  ParamDataTypeStr=Inherit: Same as input
  xmstar/xlr3 : Gain  Gain=(Xmstar/Xls)-1  SaturateOnIntegerOverflow=on  OutDataTypeStr=Inherit: Same as input  ParamDataTypeStr=Inherit: Same as input
  Fds : Outport
  wires:
  Fdr/1 -> xmstar/xlr/1
  Fqs/1 -> Product/2
  vds/1 -> Sum/1
  we/1 -> wb/1
  xmstar/xlr3/1 -> Sum1/2
  Integrator/1 -> Fds/1, xmstar/xlr3/1
  xmstar/xlr2/1 -> Integrator/1
  Sum/1 -> xmstar/xlr2/1
  xmstar/xlr1/1 -> Sum/3
  Sum1/1 -> xmstar/xlr1/1
  xmstar/xlr/1 -> Sum1/1
  Product/1 -> Sum/2
  wb/1 -> Product/1

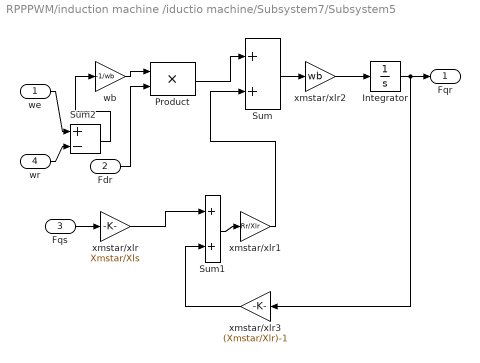
== system RPPPWM/induction machine /iductio machine/Subsystem7/Subsystem5 ==
  we : Inport
  Fdr : Inport  Port=2
  Fqs : Inport  Port=3
  wr : Inport  Port=4
  Integrator : Integrator
  Product : Product  SaturateOnIntegerOverflow=on  OutDataTypeStr=Inherit: Same as first input
  Sum : Sum  SaturateOnIntegerOverflow=on
  Sum1 : Sum  SaturateOnIntegerOverflow=on
  Sum2 : Sum  Inputs=+-  SaturateOnIntegerOverflow=on
  wb : Gain  Gain=-1/wb  SaturateOnIntegerOverflow=on  OutDataTypeStr=Inherit: Same as input  ParamDataTypeStr=Inherit: Same as input
  xmstar/xlr : Gain  Gain=Xmstar/Xls  SaturateOnIntegerOverflow=on  OutDataTypeStr=Inherit: Same as input  ParamDataTypeStr=Inherit: Same as input
  xmstar/xlr1 : Gain  Gain=Rr/Xlr  SaturateOnIntegerOverflow=on  OutDataTypeStr=Inherit: Same as input  ParamDataTypeStr=Inherit: Same as input
  xmstar/xlr2 : Gain  Gain=wb  SaturateOnIntegerOverflow=on  OutDataTypeStr=Inherit: Same as input  ParamDataTypeStr=Inherit: Same as input
  xmstar/xlr3 : Gain  Gain=(Xmstar/Xlr)-1  SaturateOnIntegerOverflow=on  OutDataTypeStr=Inherit: Same as input  ParamDataTypeStr=Inherit: Same as input
  Fqr : Outport
  wires:
  wb/1 -> Product/1
  xmstar/xlr/1 -> Sum1/1
  Sum1/1 -> xmstar/xlr1/1
  Sum/1 -> xmstar/xlr2/1
  xmstar/xlr2/1 -> Integrator/1
  Integrator/1 -> xmstar/xlr3/1, Fqr/1
  xmstar/xlr3/1 -> Sum1/2
  Fdr/1 -> Product/2
  Fqs/1 -> xmstar/xlr/1
  Product/1 -> Sum/1
  xmstar/xlr1/1 -> Sum/2
  we/1 -> Sum2/1
  wr/1 -> Sum2/2
  Sum2/1 -> wb/1

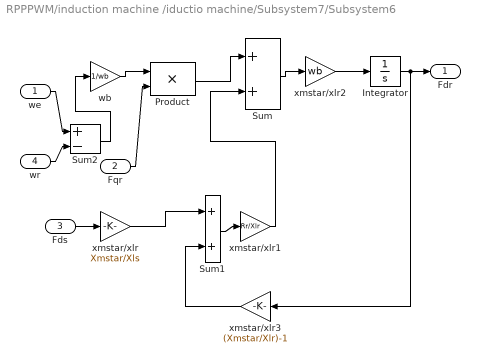
== system RPPPWM/induction machine /iductio machine/Subsystem7/Subsystem6 ==
  we : Inport
  Fqr : Inport  Port=2
  Fds : Inport  Port=3
  wr : Inport  Port=4
  Integrator : Integrator  InitialCondition=0.00001
  Product : Product  SaturateOnIntegerOverflow=on  OutDataTypeStr=Inherit: Same as first input
  Sum : Sum  SaturateOnIntegerOverflow=on
  Sum1 : Sum  SaturateOnIntegerOverflow=on
  Sum2 : Sum  Inputs=+-  SaturateOnIntegerOverflow=on
  wb : Gain  Gain=1/wb  SaturateOnIntegerOverflow=on  OutDataTypeStr=Inherit: Same as input  ParamDataTypeStr=Inherit: Same as input
  xmstar/xlr : Gain  Gain=Xmstar/Xls  SaturateOnIntegerOverflow=on  OutDataTypeStr=Inherit: Same as input  ParamDataTypeStr=Inherit: Same as input
  xmstar/xlr1 : Gain  Gain=Rr/Xlr  SaturateOnIntegerOverflow=on  OutDataTypeStr=Inherit: Same as input  ParamDataTypeStr=Inherit: Same as input
  xmstar/xlr2 : Gain  Gain=wb  SaturateOnIntegerOverflow=on  OutDataTypeStr=Inherit: Same as input  ParamDataTypeStr=Inherit: Same as input
  xmstar/xlr3 : Gain  Gain=(Xmstar/Xlr)-1  SaturateOnIntegerOverflow=on  OutDataTypeStr=Inherit: Same as input  ParamDataTypeStr=Inherit: Same as input
  Fdr : Outport
  wires:
  Sum2/1 -> wb/1
  wr/1 -> Sum2/2
  we/1 -> Sum2/1
  xmstar/xlr1/1 -> Sum/2
  Product/1 -> Sum/1
  Fds/1 -> xmstar/xlr/1
  Fqr/1 -> Product/2
  xmstar/xlr3/1 -> Sum1/2
  Integrator/1 -> Fdr/1, xmstar/xlr3/1
  xmstar/xlr2/1 -> Integrator/1
  Sum/1 -> xmstar/xlr2/1
  Sum1/1 -> xmstar/xlr1/1
  xmstar/xlr/1 -> Sum1/1
  wb/1 -> Product/1
